simulink model "Controlador PI"  (R2020a)
settings: Solver=VariableStepAuto  StartTime=0.0  StopTime=6  RelTol=1e-3
libraries: simulink x1
settings Model: Creator=danie  LastModifiedBy=danie

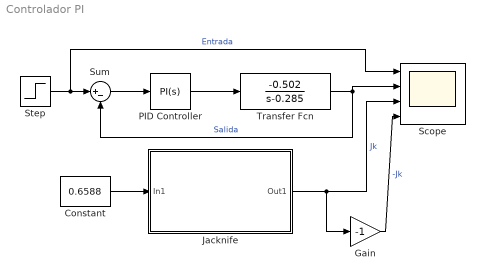
== system Controlador PI ==
  Constant : Constant  Value=0.6588
  Gain : Gain  Gain=-1
  Jacknife : Subsystem
  PID Controller : simulink/Continuous/PID Controller  Controller=PI  Form=Parallel  TimeDomain=Continuous-time  UseExternalTs=off  SampleTime=-1  IntegratorMethod=Forward Euler  FilterMethod=Forward Euler  ControllerParametersSource=internal  P=-16.5  I=-46.61  D=0  UseFilter=on  N=100  TunerSelectOption=Transfer Function Based (PID Tuner App)  InitialConditionSource=internal  InitialConditionForIntegrator=0  InitialConditionForFilter=0  DifferentiatorICPrevScaledInput=0  ExternalReset=none  TrackingMode=off  Kt=1  LimitOutput=on  UpperSaturationLimit=0.59  LowerSaturationLimit=-0.59  LinearizeAsGain=on  AntiWindupMode=back-calculation  Kb=4  POutMin=[]  POutMax=[]  IOutMin=[]  IOutMax=[]  DOutMin=[]  DOutMax=[]  NOutMin=[]  NOutMax=[]  SumOutMin=[]  SumOutMax=[]  SaturationOutMin=[]  SaturationOutMax=[]  PParamMin=[]  PParamMax=[]  IParamMin=[]  IParamMax=[]  DParamMin=[]  DParamMax=[]  NParamMin=[]  NParamMax=[]  KbParamMin=[]  KbParamMax=[]  KtParamMin=[]  KtParamMax=[]  KbOutMin=[]  KbOutMax=[]  KtOutMin=[]  KtOutMax=[]  IntegratorOutMin=[]  IntegratorOutMax=[]  FilterOutMin=[]  FilterOutMax=[]  SumI1OutMin=[]  SumI1OutMax=[]  SumI2OutMin=[]  SumI2OutMax=[]  SumI3OutMin=[]  SumI3OutMax=[]  SumI4OutMin=[]  SumI4OutMax=[]  SumDOutMin=[]  SumDOutMax=[]  DifferentiatorOutMin=[]  DifferentiatorOutMax=[]  FilterDiffOutCoefMin=[]  FilterDiffOutCoefMax=[]  ReciprocalOutMin=[]  ReciprocalOutMax=[]  SumDenOutMin=[]  SumDenOutMax=[]  SumNumOutMin=[]  SumNumOutMax=[]  DivideOutMin=[]  DivideOutMax=[]  UdiffTsProdOutMin=[]  UdiffTsProdOutMax=[]  NTsProdOutMin=[]  NTsProdOutMax=[]  UintegralTsProdOutMin=[]  UintegralTsProdOutMax=[]  UngainTsProdOutMin=[]  UngainTsProdOutMax=[]  IntegratorContinuousStateAttributes=''  IntegratorStateMustResolveToSignalObject=off  IntegratorRTWStateStorageClass=Auto  FilterContinuousStateAttributes=''  FilterStateMustResolveToSignalObject=off  FilterRTWStateStorageClass=Auto  ParallelPVariant=InternalParameters  IdealPVariant=Disabled  IVariant=InternalParameters  DVariant=Disabled  IntegratorVariant=Continuous  SatVariant=Enabled  AWVariant=BackCalculation  PCopyVariant=Disabled  TRVariant=Disabled  FdbkBlocksVariant=Forward  IdealPFdbkVariant=Disabled  SatFdbkVariant=Disabled  DerivativeFilterVariant=Disabled  NVariant=Disabled  NCopyVariant=Disabled_SignalSpec  FilterICVariant=Disabled  IntegratorICVariant=InternalICs  ExternalResetVariant=Disabled  TRSumVariant=Passthrough  SumFdbkVariant=Disabled  SumVariant=Sum_PI  TsampFilterVariant=InternalTs  TsampNgainVariant=Passthrough  TsampIntegralVariant=Passthrough
  Scope : Scope  NumInputPorts=4
  Step : Step  Time=0  After=0.78  SampleTime=0
  Sum : Sum  Inputs=|+-
  Transfer Fcn : TransferFcn  Numerator=[-0.502]  Denominator=[1 -0.285]
  wires:
  PID Controller/1 -> Transfer Fcn/1
  Transfer Fcn/1 -> Sum/2, Scope/2  "Salida"
  Sum/1 -> PID Controller/1
  Step/1 -> Sum/1, Scope/1  "Entrada"
  Constant/1 -> Jacknife/1(In1)
  Jacknife/1(Out1) -> Gain/1, Scope/3  "Jk"
  Gain/1 -> Scope/4  "-Jk"

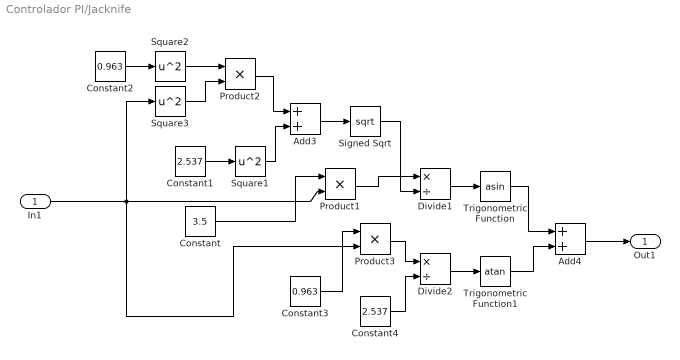
== system Controlador PI/Jacknife ==
  In1 : Inport
  Add3 : Sum
  Add4 : Sum
  Constant : Constant  Value=3.5
  Constant1 : Constant  Value=2.537
  Constant2 : Constant  Value=0.963
  Constant3 : Constant  Value=0.963
  Constant4 : Constant  Value=2.537
  Divide1 : Product  Inputs=*/
  Divide2 : Product  Inputs=*/
  Product1 : Product
  Product2 : Product
  Product3 : Product
  Signed Sqrt : Sqrt  SaturateOnIntegerOverflow=on
  Square1 : Math  Operator=square  SaturateOnIntegerOverflow=on
  Square2 : Math  Operator=square  SaturateOnIntegerOverflow=on
  Square3 : Math  Operator=square  SaturateOnIntegerOverflow=on
  Trigonometric Function : Trigonometry  Operator=asin
  Trigonometric Function1 : Trigonometry  Operator=atan
  Out1 : Outport
  wires:
  Constant1/1 -> Square1/1
  Product2/1 -> Add3/1
  Divide1/1 -> Trigonometric Function/1
  Constant2/1 -> Square2/1
  Product1/1 -> Divide1/1
  Add4/1 -> Out1/1
  Trigonometric Function1/1 -> Add4/2
  Product3/1 -> Divide2/1
  Signed Sqrt/1 -> Divide1/2
  Add3/1 -> Signed Sqrt/1
  Constant4/1 -> Divide2/2
  Square1/1 -> Add3/2
  Square2/1 -> Product2/1
  Constant/1 -> Product1/1
  Trigonometric Function/1 -> Add4/1
  Divide2/1 -> Trigonometric Function1/1
  Square3/1 -> Product2/2
  In1/1 -> Square3/1, Product1/2, Product3/2
  Constant3/1 -> Product3/1
